simulink model "test_data_type"  (R2023b)
settings: Solver=VariableStepAuto  StartTime=0.0  StopTime=10.0  RelTol=1e-3
libraries: simulink x1
settings Model: Creator=fy153  LastModifiedBy=fy153
settings OptimizationCC: DefaultUnderspecifiedDataType=single

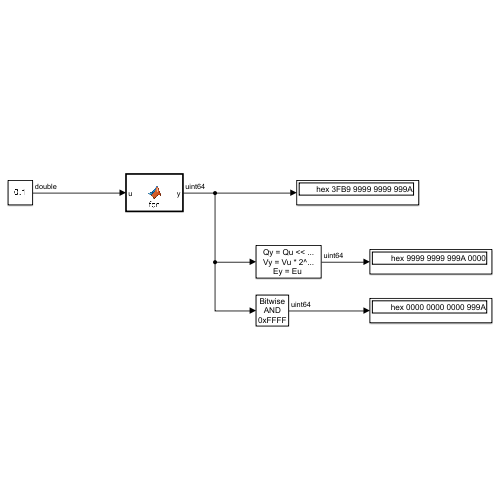
[thumbnail: Simulink's stored preview of the top-level diagram]
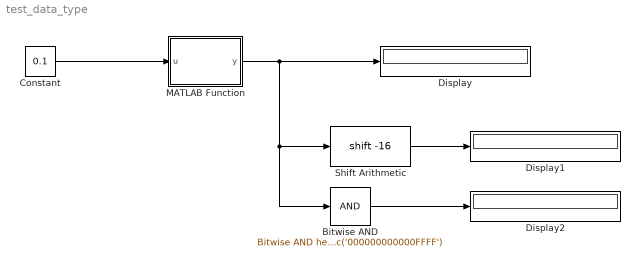
== system test_data_type ==
  Bitwise AND : simulink/Logic and Bit Operations/Bitwise Operator  logicop=AND  UseBitMask=on  BitMask=hex2dec('000000000000FFFF')  BitMaskRealWorld=Stored Integer
      settings: LibrarySourceBlock=|
      | simulink/Quick Insert/Logic and Bit
      | Operations/Bitwise AND
  Constant : Constant  Value=0.1
  Display : Display
      settings: Format=hex (Stored Integer)
  Display1 : Display
      settings: Format=hex (Stored Integer)
  Display2 : Display
      settings: Format=hex (Stored Integer)
  MATLAB Function : MATLAB Function  TreatAsAtomicUnit=on
  Shift Arithmetic : ArithShift  BitShiftNumber=-16
  wires:
  Constant/1 -> MATLAB Function/1(u)
  MATLAB Function/1(y) -> Bitwise AND/1, Shift Arithmetic/1, Display/1
  Shift Arithmetic/1 -> Display1/1
  Bitwise AND/1 -> Display2/1

== matlab function test_data_type/MATLAB Function ==
  data: u input; y output
function y = fcn(u)

y = typecast(u, 'uint64');

end
